simulink model "example1"  (Simulink 7.1)
settings: Solver=ode45  StartTime=0.0  StopTime=10.0  MaxStep=0.2  RelTol=1e-3
undefined symbols (not defined in the file or in its folder): FDab, planar
libraries: simulink x5
settings Model: Creator=roy  LastModifiedBy=roy
settings DataIOCC: LimitDataPoints=off

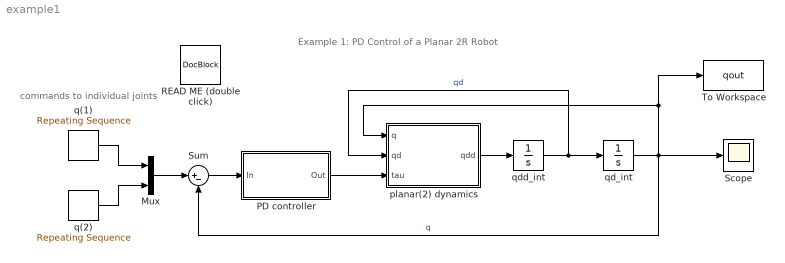
== system example1 ==
  note: Example 1: PD Control of a Planar 2R Robot
  note: commands to
      | individual
      | joints
  Mux : Mux  Inputs=2
  PD controller : Subsystem
  READ ME (double click) : simulink/Model-Wide Utilities/DocBlock  SystemSampleTime=-1  DocumentType=Text
      content=|
      | This Simulink model provides a very simple example of how to simulate a
      | robot under closed-loop control.  In this case, the robot is "planar(2)",
      | which is a two-link planar robot with revolute joints, which moves in a
      | horizontal plane (so no gravity).  The controller is a very simple
      | proportional-plus-derivative (PD) controller, which has been deliberately
      | de-tuned so as to give poor tracking accuracy, so you can see how the
      | dynamics of the robot affect the performance.
      |
      | You can run this simulation right away: just click on "start" in the
      | simulation menu, and watch the signals appear in the scope window.  (If
      | you don't have a scope window, then double-click on the scope block in
      | the model's main window.)  When the simulation is finished, you will find
      | that two new variables, called "tout" and "qout", have appeared in the
      | Matlab workspace.  Now type the command "showmotion(planar(2),tout,qout)"
      | into the Matlab command window.  This will invoke showmotion, which will
      | show you an animation of how the robot moved during the simulation.
      | Observe that showmotion is a post-processing tool: it uses recorded data
      | to show you the results of a simulation after it has finished.  Showmotion
      | cannot show you what is happening while a simulation is in progress.
      |
      | Having run the simulation and seen the result, you will probably want to
      | explore this model a bit, and maybe try some changes.  To help you do
      | this, you will find other documantation blocks in the subsystems "PD
      | controller" and "planar(2) dynamics" -- just double-click on the relevant
      | subsystem block to see what's inside.
      |
      | Tip: If you change something and re-run the simulation, then new values
      | will be stored in the Matlab variables tout and qout.  However, showmotion
      | will continue to show you the old animation until you re-issue the command
      | "showmotion(planar(2),tout,qout)".
      |
      | Before you dive into the subsystems, here is an overview of how the model
      | works.  First, a motion command signal is generated in the two blocks
      | labelled q(1) and q(2).  These signals define the commanded motions of
      | joints 1 and 2, respectively, in units of radians.  These two signals are
      | then combined to form a 2x1 column vector, which is the position command
      | signal for the whole robot.  Next, the actual position (q) is subtracted
      | from the commanded position, and the difference (the tracking error) is
      | fed to the controller.  The output of the controller specifies the joint
      | force command; that is, the 2x1 vector of torques that must be applied at
      | joints 1 and 2.  This signal is fed to the joint-force input (tau) of the
      | dynamics block, which calculates the joint accelerations (qdd) caused by
      | the applied forces.  The accelerations are then integrated twice to obtain
      | the joint velocity vector (qd) and position vector (q).  These two signals
      | are then fed back into the dynamics block because the robot's dynamics
      | depends on their values.  Finally, q is sent to a scope, so you can see
      | it, and also to the Matlab workspace variable qout.  (Simulink
      | automatically saves tout.)
      |
      | Here are some things you can try:
      |
      | 1.  You can change the motion command by altering the data in blocks q(1)
      |     and q(2).
      |
      | 2.  You can watch other signals, like qd, by adding scope blocks and
      |     connecting them to the signals of interest.
      |
      | 3.  You can plot qout vs. tout in Matlab using the following commands:
      |        tmp=[]; tmp(:,:)=qout(:,1,:);
      |        plot( tout, tmp );
      |
      | Now take a look at the subsystems "PD controller" and "planar(2)
      | dynamics".
  Scope : Scope
      settings: YMin=-0.2  YMax=2.2
  Sum : Sum  Inputs=|+-  OutDataType=sfix(16)  OutScaling=2^0
  To Workspace : ToWorkspace  VariableName=qout  SampleTime=-1  SaveFormat=Array
  planar(2) dynamics : Subsystem
  q(1) : simulink/Sources/Repeating Sequence  SystemSampleTime=-1  rep_seq_t=[0 1 2 3 4]  rep_seq_y=[0 1 1 0 0]
  q(2) : simulink/Sources/Repeating Sequence  SystemSampleTime=-1  rep_seq_t=[0 1 2 3 4]  rep_seq_y=[0 2 2 0 0]
  qd_int : Integrator
  qdd_int : Integrator
  wires:
  q(1)/1 -> Mux/1
  q(2)/1 -> Mux/2
  Mux/1 -> Sum/1
  Sum/1 -> PD controller/1(In)
  PD controller/1(Out) -> planar(2) dynamics/3(tau)
  planar(2) dynamics/1(qdd) -> qdd_int/1
  qdd_int/1 -> qd_int/1, planar(2) dynamics/2(qd)  "qd"
  qd_int/1 -> Scope/1, Sum/2, planar(2) dynamics/1(q), To Workspace/1  "q"

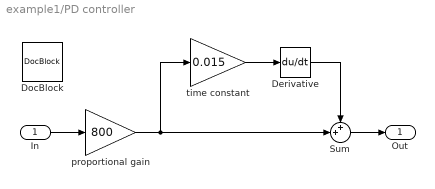
== system example1/PD controller ==
  In : Inport  OutDataType=sfix(16)  OutScaling=2^0
  Derivative : Derivative
  DocBlock : simulink/Model-Wide Utilities/DocBlock  SystemSampleTime=-1  DocumentType=Text
      content=|
      | This control system is deliberately badly tuned, so that you can see the
      | dynamics in action.  Observe that the wobbling is worse, and at a lower
      | frequency, when the robot is straight than when it is bent.  Also, it is
      | mostly joint 1 that wobbles.  These are both consequences of the dynamics:
      | the robot exhibits a larger inertia about joint 1 than about joint 2,
      | meaning that a larger force is required to make joint 1 move than joint 2.
      | Furthermore, the inertia is larger when the robot is straight than when it
      | is bent.
      |
      | Once you have seen how badly this controller works, try changing the
      | gains.  For example, increasing the proportional gain (e.g. to 1500) will
      | make an obvious improvement.  Increasing the time constant will increase
      | the damping -- try increasing it to 0.05 to see what happens.  Another
      | thing you can do is make the gains different for joints 1 and 2.  For
      | example, setting the proportional gain to [1000; 100] will apply a gain of
      | 1000 to joint 1 and 100 (which is too low) to joint 2.  Now it is joint 2
      | that does most of the wobbling.
  Sum : Sum  Inputs=++|  OutDataType=sfix(16)  OutScaling=2^0
  proportional gain : Gain  Gain=800  ParameterDataType=sfix(16)  ParameterScaling=2^0  OutDataType=sfix(16)  OutScaling=2^0
  time constant : Gain  Gain=0.015  ParameterDataType=sfix(16)  ParameterScaling=2^0  OutDataType=sfix(16)  OutScaling=2^0
  Out : Outport  OutDataType=sfix(16)  OutScaling=2^0
  wires:
  In/1 -> proportional gain/1
  proportional gain/1 -> Sum/2, time constant/1
  time constant/1 -> Derivative/1
  Derivative/1 -> Sum/1
  Sum/1 -> Out/1

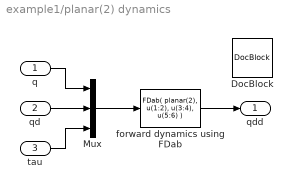
== system example1/planar(2) dynamics ==
  q : Inport  OutDataType=sfix(16)  OutScaling=2^0
  qd : Inport  Port=2  OutDataType=sfix(16)  OutScaling=2^0
  tau : Inport  Port=3  OutDataType=sfix(16)  OutScaling=2^0
  DocBlock : simulink/Model-Wide Utilities/DocBlock  SystemSampleTime=-1  DocumentType=Text
      content=|
      | This subsystem shows the simplest method for incorporating dynamics
      | calculations into a Simulink model.  Simulink provides a "MATLAB function"
      | block, to allow Matlab functions to be incorporated into a Simulink model.
      | However, this block has only a single input and a single output.
      | Therefore, the first thing that must happen is that the three variables
      | needed for the dynamics calculation (q, qd and tau) must be combined into
      | a single vector, so that it can be fed in as the single input to the
      | Matlab function block.  If you open this block, you will find that the
      | actual function call is "FDab( planar(2), u(1:2), u(3:4), u(5:6) )".  The
      | expressions u(1:2), u(3:4) and u(5:6) extract the 2x1 vectors q, qd and
      | tau from the 6x1 input vector u, so that the call is effectively
      | "FDab( planar(2), q, qd, tau )".
      |
      | There is one more important thing to note about this block: Simulink needs
      | to be told the type and dimensions of the return value.  Now, the return
      | value (qdd) is a 2x1 vector of real numbers (because planar(2) has two
      | joint variables); so the Matlab function block's parameter "Output
      | dimensions:" has to be set to "[2 1]", the output signal type must be set
      | to "real", and the box "Collapse 2-D results to 1-D" must be un-checked.
      |
      | "planar(2)" is a call to the model-creating function "planar".  This
      | function will be called every time that FDab is called, which is several
      | times per integration step.  If planar were to create a new model every
      | time it was called, it would be an obvious piece of inefficiency.
      | However, if you look at the source code of planar (in models/planar.m),
      | you will find that it stores a copy of the last model it made, and returns
      | that copy if the argument matches.
      |
      | This style of use, in which a dynamics function (like FDab) is called
      | directly, the input vector u is explicitly split into its component parts,
      | and a model-preparation function (like planar) supplies a model at every
      | call, is the simplest way to proceed.  The only snags are: (1) you need to
      | get the numbers right, and (2) for the sake of efficiency, the
      | model-preparation function ought to use the same strategy that you see in
      | planar.  If you wanted to modify this Simulink model to use planar(3)
      | (i.e., a three-joint robot) instead of planar(2), then you would have to
      | change the function call to read
      | "FDab( planar(3), u(1:3), u(4:6), u(7:9) )", and you would have to change
      | the output dimensions to "[3 1]".  You would also have to supply a motion
      | command signal for q(3).
  Mux : Mux  Inputs=3
  forward dynamics using FDab : MATLABFcn  MATLABFcn=FDab( planar(2), u(1:2), u(3:4), u(5:6) )  OutputDimensions=[2 1]  OutputSignalType=real  Output1D=off
  qdd : Outport  OutDataType=sfix(16)  OutScaling=2^0
  wires:
  qd/1 -> Mux/2
  q/1 -> Mux/1
  tau/1 -> Mux/3
  Mux/1 -> forward dynamics using FDab/1
  forward dynamics using FDab/1 -> qdd/1
